simulink model "OutputAdaptive"  (R2022b)
settings: Solver=VariableStepAuto  StartTime=0.0  StopTime=100  RelTol=1e-3
values from neighbouring files (symbols this model uses):
  a0 = 0    [consts.m]
  a1 = 0    [consts.m]
  b0 = 1    [consts.m]
  b1 = 0    [consts.m]
  dy0 = 0    [consts.m]
  e = [1]    [consts.m]
  g = 1    [consts.m]
  gamma = 0.5    [consts.m]
  k0 = 1    [consts.m]
  km0 = 1    [consts.m]
  km1 = 2    [consts.m]
  km2 = 1    [consts.m]
  LAM = [-k0]    [consts.m]
  y0 = 5    [consts.m]
settings Model: Creator=zein  LastModifiedBy=zein

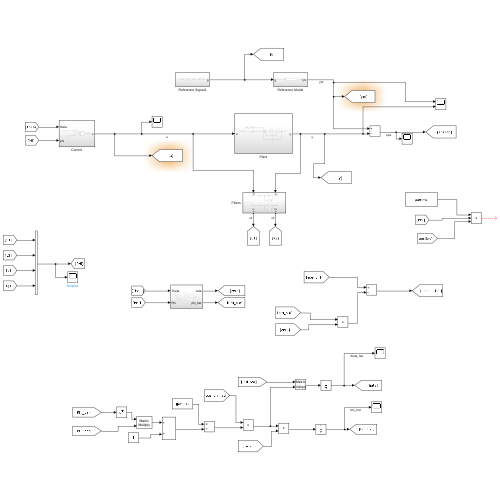
[thumbnail: Simulink's stored preview of the top-level diagram]
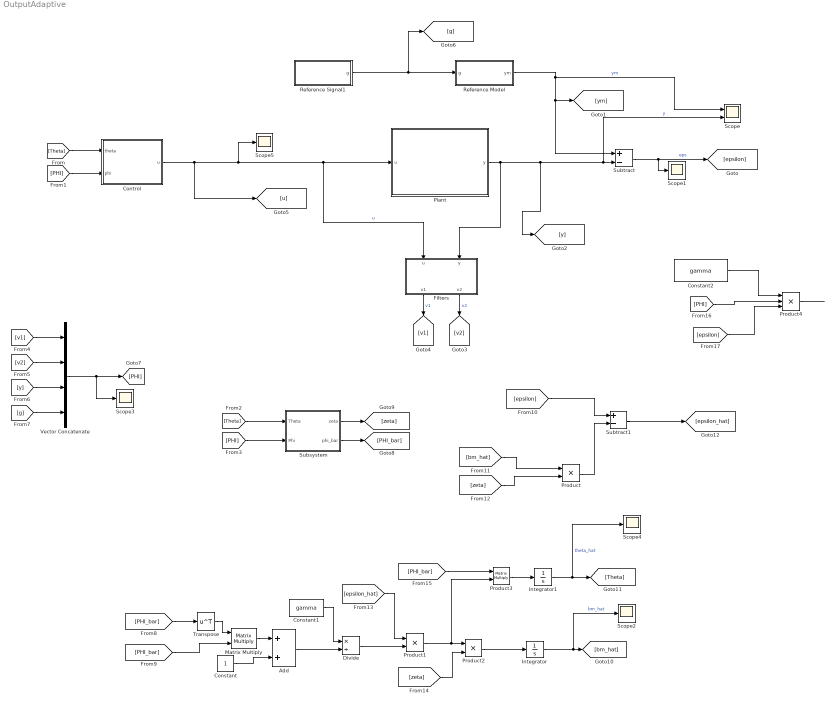
== system OutputAdaptive ==
  Add : Sum
  Constant : Constant
  Constant1 : Constant  Value=gamma
  Constant2 : Constant  Value=gamma
  Control : Subsystem
  Divide : Product  Inputs=*/
  Filters : Subsystem
  Integrator : Integrator
  Integrator1 : Integrator
  Matrix Multiply : Product  Multiplication=Matrix(*)
  Plant : Subsystem
  Product : Product
  Product1 : Product
  Product2 : Product
  Product3 : Product  Multiplication=Matrix(*)
  Product4 : Product  Inputs=3
  Reference Model : Subsystem
  Reference Signal1 : Subsystem
  Scope : Scope  NumInputPorts=2
  Scope{1..5} (5 alike) : Scope
  Subsystem : Subsystem
  Subtract : Sum  Inputs=+-
  Subtract1 : Sum  Inputs=+-
  Transpose : Math  Operator=transpose
  Vector Concatenate : Concatenate  NumInputs=4  Mode=Multidimensional array
  wires:
  Control/1(u) -> [u], Scope5/1, Filters/1(u), Plant/1(u)  "u"
  Plant/1(y) -> [y], Scope/2, Subtract/2, Filters/2(y)  "y"
  Reference Signal1/1(g) -> [g], Reference Model/1(g)
  Reference Model/1(ym) -> Scope/1, Subtract/1, [ym]  "ym"
  Subtract/1 -> Scope1/1, [epsilon]  "eps"
  Filters/2(v2) -> [v2]  "v2"
  Filters/1(v1) -> [v1]  "v1"
  [Theta] -> Control/1(theta)
  [PHI] -> Control/2(phi)
  [Theta] -> Subsystem/1(Theta)
  [PHI] -> Subsystem/2(Phi)
  [v1] -> Vector Concatenate/1
  [v2] -> Vector Concatenate/2
  [y] -> Vector Concatenate/3
  [g] -> Vector Concatenate/4
  Subsystem/1(zeta) -> [zeta]
  Subsystem/2(phi_bar) -> [PHI_bar]
  Integrator/1 -> Scope2/1, [bm_hat]  "bm_hat"
  Integrator1/1 -> [Theta], Scope4/1  "theta_hat"
  [PHI_bar] -> Transpose/1
  Transpose/1 -> Matrix Multiply/1
  [PHI_bar] -> Matrix Multiply/2
  Matrix Multiply/1 -> Add/1
  Constant/1 -> Add/2
  Add/1 -> Divide/2
  Constant1/1 -> Divide/1
  [epsilon] -> Subtract1/1
  [bm_hat] -> Product/1
  [zeta] -> Product/2
  Product/1 -> Subtract1/2
  Subtract1/1 -> [epsilon_hat]
  Divide/1 -> Product1/2
  [epsilon_hat] -> Product1/1
  Product1/1 -> Product3/2, Product2/1
  [zeta] -> Product2/2
  Product2/1 -> Integrator/1
  Product3/1 -> Integrator1/1
  [PHI_bar] -> Product3/1
  Vector Concatenate/1 -> Scope3/1, [PHI]
  Product4/1 -> ?
  [epsilon] -> Product4/3
  [PHI] -> Product4/2
  Constant2/1 -> Product4/1

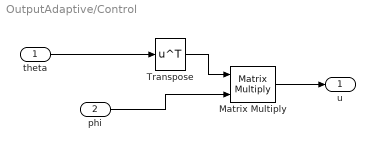
== system OutputAdaptive/Control ==
  theta : Inport
  phi : Inport  Port=2
  Matrix Multiply : Product  Multiplication=Matrix(*)
  Transpose : Math  Operator=transpose
  u : Outport
  wires:
  theta/1 -> Transpose/1
  Transpose/1 -> Matrix Multiply/1
  phi/1 -> Matrix Multiply/2
  Matrix Multiply/1 -> u/1

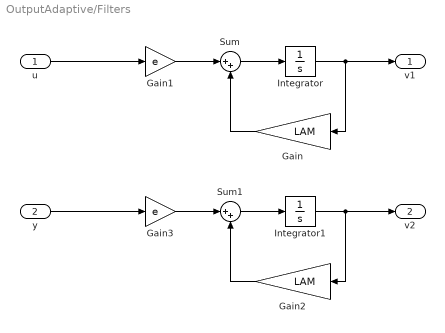
== system OutputAdaptive/Filters ==
  u : Inport
  y : Inport  Port=2
  Gain : Gain  Gain=LAM
  Gain1 : Gain  Gain=e
  Gain2 : Gain  Gain=LAM
  Gain3 : Gain  Gain=e
  Integrator : Integrator
  Integrator1 : Integrator  InitialCondition=y0
  Sum : Sum  Inputs=|++
  Sum1 : Sum  Inputs=|++
  v1 : Outport
  v2 : Outport  Port=2
  wires:
  Gain2/1 -> Sum1/2
  Sum/1 -> Integrator/1
  Gain1/1 -> Sum/1
  u/1 -> Gain1/1
  Gain/1 -> Sum/2
  Gain3/1 -> Sum1/1
  Sum1/1 -> Integrator1/1
  Integrator/1 -> v1/1, Gain/1
  y/1 -> Gain3/1
  Integrator1/1 -> v2/1, Gain2/1

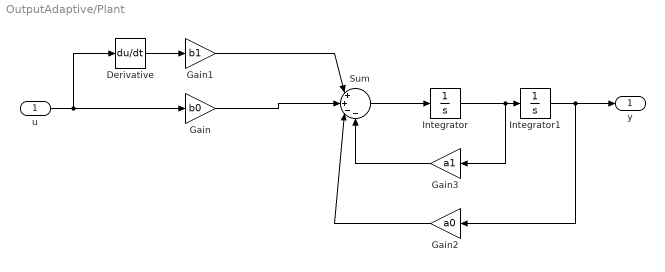
== system OutputAdaptive/Plant ==
  u : Inport
  Derivative : Derivative  CoefficientInTFapproximation=0
  Gain : Gain  Gain=b0
  Gain1 : Gain  Gain=b1
  Gain2 : Gain  Gain=a0
  Gain3 : Gain  Gain=a1
  Integrator : Integrator  InitialCondition=dy0
  Integrator1 : Integrator  InitialCondition=y0
  Sum : Sum  Inputs=|++--
  y : Outport
  wires:
  Integrator/1 -> Gain3/1, Integrator1/1
  Integrator1/1 -> Gain2/1, y/1
  u/1 -> Derivative/1, Gain/1
  Derivative/1 -> Gain1/1
  Sum/1 -> Integrator/1
  Gain1/1 -> Sum/1
  Gain/1 -> Sum/2
  Gain3/1 -> Sum/4
  Gain2/1 -> Sum/3

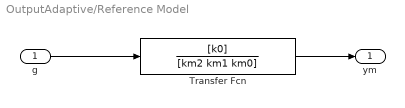
== system OutputAdaptive/Reference Model ==
  g : Inport
  Transfer Fcn : TransferFcn  Numerator=[k0]  Denominator=[km2 km1 km0]
  ym : Outport
  wires:
  g/1 -> Transfer Fcn/1
  Transfer Fcn/1 -> ym/1

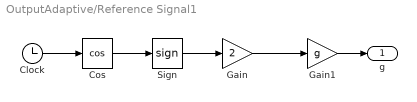
== system OutputAdaptive/Reference Signal1 ==
  Clock : Clock
  Cos : Trigonometry  Operator=cos
  Gain : Gain  Gain=2
  Gain1 : Gain  Gain=g
  Sign : Signum
  g : Outport
  wires:
  Cos/1 -> Sign/1
  Sign/1 -> Gain/1
  Clock/1 -> Cos/1
  Gain/1 -> Gain1/1
  Gain1/1 -> g/1

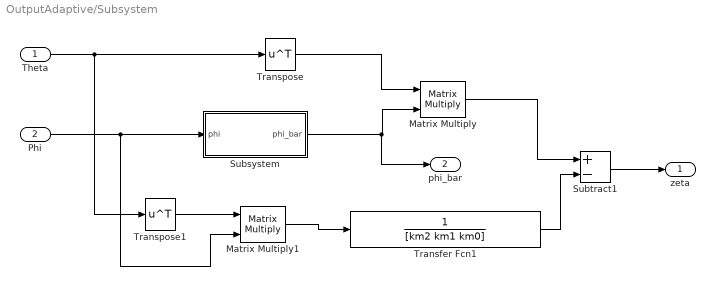
== system OutputAdaptive/Subsystem ==
  Theta : Inport
  Phi : Inport  Port=2
  Matrix Multiply : Product  Multiplication=Matrix(*)
  Matrix Multiply1 : Product  Multiplication=Matrix(*)
  Subsystem : Subsystem
  Subtract1 : Sum  Inputs=+-
  Transfer Fcn1 : TransferFcn  Denominator=[km2 km1 km0]
  Transpose : Math  Operator=transpose
  Transpose1 : Math  Operator=transpose
  zeta : Outport
  phi_bar : Outport  Port=2
  wires:
  Subsystem/1(phi_bar) -> phi_bar/1, Matrix Multiply/2
  Matrix Multiply/1 -> Subtract1/1
  Transpose/1 -> Matrix Multiply/1
  Transpose1/1 -> Matrix Multiply1/1
  Theta/1 -> Transpose1/1, Transpose/1
  Subtract1/1 -> zeta/1
  Matrix Multiply1/1 -> Transfer Fcn1/1
  Transfer Fcn1/1 -> Subtract1/2
  Phi/1 -> Subsystem/1(phi), Matrix Multiply1/2

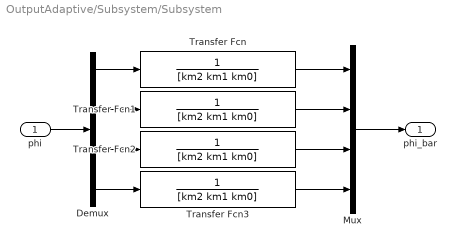
== system OutputAdaptive/Subsystem/Subsystem ==
  phi : Inport
  Demux : Demux
  Mux : Mux
  Transfer Fcn{,1..3} (4 alike) : TransferFcn  Denominator=[km2 km1 km0]
  phi_bar : Outport
  wires:
  phi/1 -> Demux/1
  Demux/1 -> Transfer Fcn/1
  Demux/2 -> Transfer Fcn1/1
  Demux/3 -> Transfer Fcn2/1
  Demux/4 -> Transfer Fcn3/1
  Mux/1 -> phi_bar/1
  Transfer Fcn3/1 -> Mux/4
  Transfer Fcn2/1 -> Mux/3
  Transfer Fcn1/1 -> Mux/2
  Transfer Fcn/1 -> Mux/1
